simulink model "gm_HDL_pfc_gold_fi_vnl"  (R2024b)
settings: Solver=FixedStepDiscrete  StartTime=0.0  StopTime=.06  RelTol=1e-3
InitFcn:
  | fidelity_pfc_vals;
  | load('C:\Users\angro\Desktop\hil\pfc3ph\matlab\sim\sschdl\pfc_desktop\stateSpaceParameters.mat');
undefined symbols (not defined in the file or in its folder): a, b, c, DiscIntNeverNeededParam, fsw, Gs, s, stateSpaceParameters_1, t_ss, tsw
libraries: simulink x55, hdlmdlgenlib x26, hdlsllib x10, mcbcontrolslib x5, dspsrcs4 x3, slpidlib x2, hdlssclib x2, spsSVPWMGenerator2LevelLib x1, spsPLL3phLib x1
(part 1 of 4)
settings Model: Creator=angro  LastModifiedBy=angro
settings OptimizationCC: BlockReduction=off  ConditionallyExecuteInputs=off  DefaultParameterBehavior=Inlined  InheritOutputTypeSmallerThanSingle=on
settings DebuggingCC: SignalRangeChecking=warning  AlgebraicLoopMsg=error  ArtificialAlgebraicLoopMsg=error  InheritedTsInSrcMsg=none  SingleTaskRateTransMsg=error  UnconnectedInputMsg=warning  UnconnectedOutputMsg=warning  UnconnectedLineMsg=warning
settings HardwareCC: ProdBitPerPointer=32  ProdBitPerSizeT=32  ProdBitPerPtrDiffT=32  ProdLargestAtomicFloat=None  ProdIntDivRoundTo=Undefined  ProdEndianess=Unspecified  ProdWordSize=32  ProdHWDeviceType=ASIC/FPGA->ASIC/FPGA  TargetBitPerPointer=64  TargetBitPerSizeT=64  TargetBitPerPtrDiffT=64  TargetLongLongMode=on  TargetIntDivRoundTo=Zero  TargetEndianess=LittleEndian  TargetWordSize=64  TargetHWDeviceType=Custom Processor->MATLAB Host Computer  ProdEqTarget=off

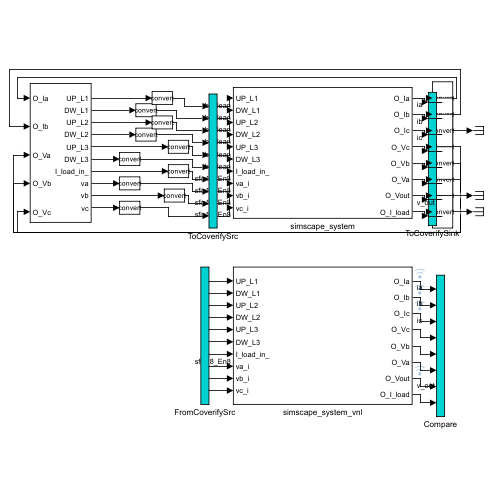
[thumbnail: Simulink's stored preview of the top-level diagram]
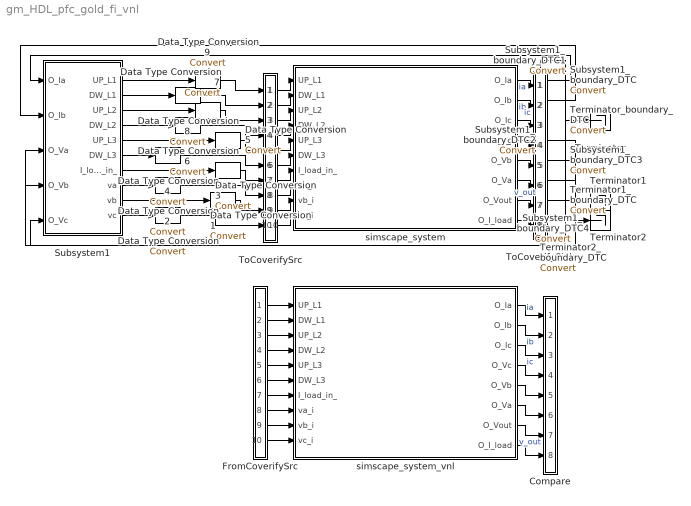
== system gm_HDL_pfc_gold_fi_vnl ==
  Compare : Subsystem
      mask Display: disp('')
  Data Type Conversion{,1..9} (10 alike) : DataTypeConversion  SaturateOnIntegerOverflow=off  RndMeth=Floor
  FromCoverifySrc : Subsystem
      mask Display: disp('')
  Subsystem1 : Subsystem
  Subsystem1_boundary_DTC{,1..4} (5 alike) : DataTypeConversion
  Terminator : Terminator
  Terminator1 : Terminator
  Terminator1_boundary_DTC : DataTypeConversion
  Terminator2 : Terminator
  Terminator2_boundary_DTC : DataTypeConversion
  Terminator_boundary_DTC : DataTypeConversion
  ToCoverifySink : Subsystem
      mask Display: disp('')
  ToCoverifySrc : Subsystem
      mask Display: disp('')
  simscape_system : Subsystem
  simscape_system_vnl : Subsystem
  wires:
  Subsystem1/7(I_load_in_) -> Data Type Conversion3/1
  Subsystem1/1(UP_L1) -> Data Type Conversion9/1
  Subsystem1/2(DW_L1) -> Data Type Conversion8/1
  Subsystem1/3(UP_L2) -> Data Type Conversion7/1
  Subsystem1/4(DW_L2) -> Data Type Conversion6/1
  Subsystem1/5(UP_L3) -> Data Type Conversion5/1
  Subsystem1/6(DW_L3) -> Data Type Conversion4/1
  Subsystem1/8(va) -> Data Type Conversion2/1
  Subsystem1/9(vb) -> Data Type Conversion1/1
  Subsystem1/10(vc) -> Data Type Conversion/1
  Subsystem1_boundary_DTC/1 -> Subsystem1/1(O_Ia)
  Subsystem1_boundary_DTC1/1 -> Subsystem1/2(O_Ib)
  Terminator_boundary_DTC/1 -> Terminator/1
  Subsystem1_boundary_DTC2/1 -> Subsystem1/5(O_Vc)
  Subsystem1_boundary_DTC3/1 -> Subsystem1/4(O_Vb)
  Subsystem1_boundary_DTC4/1 -> Subsystem1/3(O_Va)
  Terminator1_boundary_DTC/1 -> Terminator1/1
  Terminator2_boundary_DTC/1 -> Terminator2/1
  ToCoverifySrc/1(out1) -> simscape_system/1(UP_L1)
  ToCoverifySrc/2(out2) -> simscape_system/2(DW_L1)
  ToCoverifySrc/3(out3) -> simscape_system/3(UP_L2)
  ToCoverifySrc/4(out4) -> simscape_system/4(DW_L2)
  ToCoverifySrc/5(out5) -> simscape_system/5(UP_L3)
  ToCoverifySrc/6(out6) -> simscape_system/6(DW_L3)
  ToCoverifySrc/7(out7) -> simscape_system/7(I_load_in_)
  ToCoverifySrc/8(out8) -> simscape_system/8(va_i)
  ToCoverifySrc/9(out9) -> simscape_system/9(vb_i)
  ToCoverifySrc/10(out10) -> simscape_system/10(vc_i)
  simscape_system/1(O_Ia) -> ToCoverifySink/1(in1)  "ia"
  simscape_system/2(O_Ib) -> ToCoverifySink/2(in2)  "ib"
  simscape_system/3(O_Ic) -> ToCoverifySink/3(in3)  "ic"
  simscape_system/4(O_Vc) -> ToCoverifySink/4(in4)
  simscape_system/5(O_Vb) -> ToCoverifySink/5(in5)
  simscape_system/6(O_Va) -> ToCoverifySink/6(in6)
  simscape_system/7(O_Vout) -> ToCoverifySink/7(in7)  "v_out"
  simscape_system/8(O_I_load) -> ToCoverifySink/8(in8)
  Data Type Conversion9/1 -> ToCoverifySrc/1(in1)
  Data Type Conversion8/1 -> ToCoverifySrc/2(in2)
  Data Type Conversion7/1 -> ToCoverifySrc/3(in3)
  Data Type Conversion6/1 -> ToCoverifySrc/4(in4)
  Data Type Conversion5/1 -> ToCoverifySrc/5(in5)
  Data Type Conversion4/1 -> ToCoverifySrc/6(in6)
  Data Type Conversion3/1 -> ToCoverifySrc/7(in7)
  Data Type Conversion2/1 -> ToCoverifySrc/8(in8)
  Data Type Conversion1/1 -> ToCoverifySrc/9(in9)
  Data Type Conversion/1 -> ToCoverifySrc/10(in10)
  ToCoverifySink/1(out1) -> Subsystem1_boundary_DTC/1
  ToCoverifySink/2(out2) -> Subsystem1_boundary_DTC1/1
  ToCoverifySink/3(out3) -> Terminator_boundary_DTC/1
  ToCoverifySink/4(out4) -> Subsystem1_boundary_DTC2/1
  ToCoverifySink/5(out5) -> Subsystem1_boundary_DTC3/1
  ToCoverifySink/6(out6) -> Subsystem1_boundary_DTC4/1
  ToCoverifySink/7(out7) -> Terminator1_boundary_DTC/1
  ToCoverifySink/8(out8) -> Terminator2_boundary_DTC/1
  FromCoverifySrc/1(out1) -> simscape_system_vnl/1(UP_L1)
  FromCoverifySrc/2(out2) -> simscape_system_vnl/2(DW_L1)
  FromCoverifySrc/3(out3) -> simscape_system_vnl/3(UP_L2)
  FromCoverifySrc/4(out4) -> simscape_system_vnl/4(DW_L2)
  FromCoverifySrc/5(out5) -> simscape_system_vnl/5(UP_L3)
  FromCoverifySrc/6(out6) -> simscape_system_vnl/6(DW_L3)
  FromCoverifySrc/7(out7) -> simscape_system_vnl/7(I_load_in_)
  FromCoverifySrc/8(out8) -> simscape_system_vnl/8(va_i)
  FromCoverifySrc/9(out9) -> simscape_system_vnl/9(vb_i)
  FromCoverifySrc/10(out10) -> simscape_system_vnl/10(vc_i)
  simscape_system_vnl/1(O_Ia) -> Compare/1(in1)  "ia"
  simscape_system_vnl/2(O_Ib) -> Compare/2(in2)  "ib"
  simscape_system_vnl/3(O_Ic) -> Compare/3(in3)  "ic"
  simscape_system_vnl/4(O_Vc) -> Compare/4(in4)
  simscape_system_vnl/5(O_Vb) -> Compare/5(in5)
  simscape_system_vnl/6(O_Va) -> Compare/6(in6)
  simscape_system_vnl/7(O_Vout) -> Compare/7(in7)  "v_out"
  simscape_system_vnl/8(O_I_load) -> Compare/8(in8)

== system gm_HDL_pfc_gold_fi_vnl/Compare ==
  in1 : Inport
  in2 : Inport  Port=2
  in3 : Inport  Port=3
  in4 : Inport  Port=4
  in5 : Inport  Port=5
  in6 : Inport  Port=6
  in7 : Inport  Port=7
  in8 : Inport  Port=8
  Assert_O_I_load : Subsystem
  Assert_O_Ia : Subsystem
  Assert_O_Ib : Subsystem
  Assert_O_Ic : Subsystem
  Assert_O_Va : Subsystem
  Assert_O_Vb : Subsystem
  Assert_O_Vc : Subsystem
  Assert_O_Vout : Subsystem
  CleanupScopes : Subsystem
      settings: OpenFcn=|
      | blkName = gcb; %self block
      | idx = regexp(blkName, '/CleanupScopes$', 'once');
      | blkParent = blkName(1:idx-1);
      | blks=find_system(blkParent, 'LookUnderMasks', 'all','blocktype', 'Scope');
      | for itr = 1:length(blks)
      | 	 hScopeCfg = get_param(blks{itr},'ScopeConfiguration');
      | 	 hScopeCfg.Visible = ~ hScopeCfg.Visible;
      | end
      | drawnow;
      mask Display: fprintf(message('hdlcoder:cosim:vnl_dblclick').getString());
  Enable : Subsystem
      settings: OpenFcn=|
      | blkName = gcb;
      | idx = regexp(blkName, '/Enable$', 'once');
      | blkParent = blkName(1:idx-1);
      | blks=find_system(blkParent, 'LookUnderMasks', 'all','blocktype', 'Assertion');
      | e = get_param(blks{1}, 'Enabled');
      | if strcmp(e, 'on'), f= 'off';, else, f = 'on';, end
      | for ii=1:length(blks), set_param(blks{ii}, 'Enabled', f);, end
      | set_param(gcb, 'MaskDisplay',['fprintf(message(''hdlcoder:cosim:vnl_dblclick_assertions'',','''',upper(e),'''',').getString())']);
      mask Display: fprintf(message('hdlcoder:cosim:vnl_dblclick_assertions','OFF').getString());
  pathdelay{1..8} (8 alike) : Delay  DelayLength=1
  wires:
  in1/1 -> pathdelay1/1
  pathdelay1/1 -> Assert_O_Ia/1(cosim)
  [out1] -> Assert_O_Ia/2(dut)
  in2/1 -> pathdelay2/1
  pathdelay2/1 -> Assert_O_Ib/1(cosim)
  [out2] -> Assert_O_Ib/2(dut)
  in3/1 -> pathdelay3/1
  pathdelay3/1 -> Assert_O_Ic/1(cosim)
  [out3] -> Assert_O_Ic/2(dut)
  in4/1 -> pathdelay4/1
  pathdelay4/1 -> Assert_O_Vc/1(cosim)
  [out4] -> Assert_O_Vc/2(dut)
  in5/1 -> pathdelay5/1
  pathdelay5/1 -> Assert_O_Vb/1(cosim)
  [out5] -> Assert_O_Vb/2(dut)
  in6/1 -> pathdelay6/1
  pathdelay6/1 -> Assert_O_Va/1(cosim)
  [out6] -> Assert_O_Va/2(dut)
  in7/1 -> pathdelay7/1
  pathdelay7/1 -> Assert_O_Vout/1(cosim)
  [out7] -> Assert_O_Vout/2(dut)
  in8/1 -> pathdelay8/1
  pathdelay8/1 -> Assert_O_I_load/1(cosim)
  [out8] -> Assert_O_I_load/2(dut)

== system gm_HDL_pfc_gold_fi_vnl/FromCoverifySrc ==
  out1 : Outport
  out2 : Outport  Port=2
  out3 : Outport  Port=3
  out4 : Outport  Port=4
  out5 : Outport  Port=5
  out6 : Outport  Port=6
  out7 : Outport  Port=7
  out8 : Outport  Port=8
  out9 : Outport  Port=9
  out10 : Outport  Port=10
  wires:
  [in1] -> out1/1
  [in2] -> out2/1
  [in3] -> out3/1
  [in4] -> out4/1
  [in5] -> out5/1
  [in6] -> out6/1
  [in7] -> out7/1
  [in8] -> out8/1
  [in9] -> out9/1
  [in10] -> out10/1

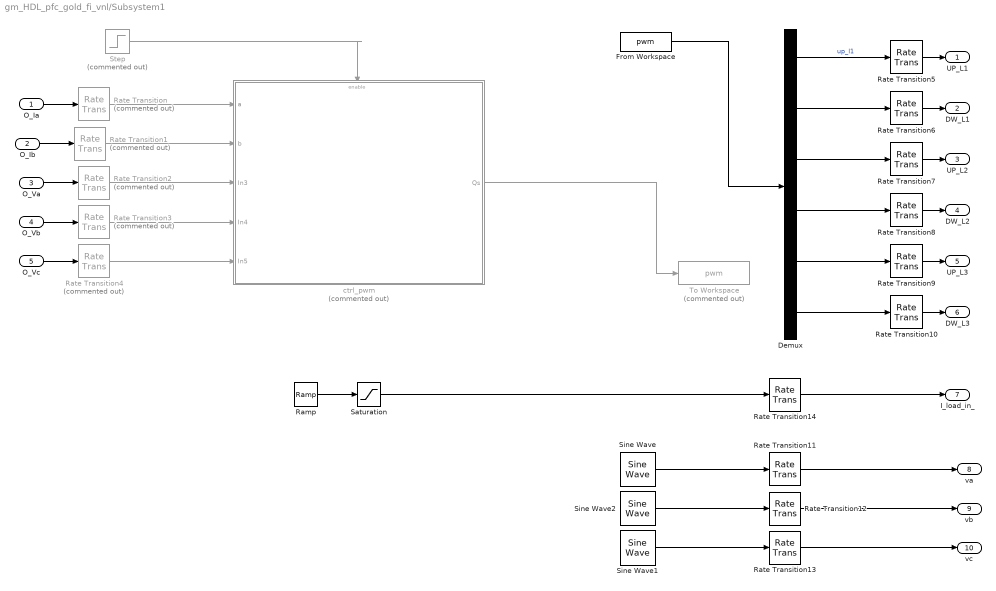
== system gm_HDL_pfc_gold_fi_vnl/Subsystem1 ==
  O_Ia : Inport
  O_Ib : Inport  Port=2
  O_Va : Inport  Port=3
  O_Vb : Inport  Port=4
  O_Vc : Inport  Port=5
  Demux : Demux  Outputs=6
  From Workspace : FromWorkspace  VariableName=pwm  SampleTime=t_ss  Interpolate=off  ZeroCross=off  OutputAfterFinalValue=Holding final value
  Ramp : simulink/Sources/Ramp  slope=1/50  start=2/50  InitialOutput=0
  Rate Transition{,1..4} (5 alike) : RateTransition  Commented=on  OutPortSampleTime=t_ss
  Rate Transition{5..10,14} (7 alike) : RateTransition  OutPortSampleTime=t_ss
  Rate Transition11 : RateTransition
  Rate Transition12 : RateTransition
  Rate Transition13 : RateTransition
  Saturation : Saturate  UpperLimit=2
  Sine Wave : dspsrcs4/Sine Wave  Amplitude=325  Frequency=50  Phase=0  SampleMode=Discrete  OutComplex=Real  CompMethod=Table lookup  TableSize=Speed  SampleTime=tsw  SamplesPerFrame=1  ResetState=Restart at time zero  OutputFrames=off  dataType=double  wordLen=16  udDataType=sfix(16)  fracBitsMode=Best precision  numFracBits=15  OutDataTypeStr=double  LastOutDataTypeStr=double
  Sine Wave1 : dspsrcs4/Sine Wave  Amplitude=325  Frequency=50  Phase=2*pi/3  SampleMode=Discrete  OutComplex=Real  CompMethod=Table lookup  TableSize=Speed  SampleTime=tsw  SamplesPerFrame=1  ResetState=Restart at time zero  OutputFrames=off  dataType=double  wordLen=16  udDataType=sfix(16)  fracBitsMode=Best precision  numFracBits=15  OutDataTypeStr=double  LastOutDataTypeStr=double
  Sine Wave2 : dspsrcs4/Sine Wave  Amplitude=325  Frequency=50  Phase=-2*pi/3  SampleMode=Discrete  OutComplex=Real  CompMethod=Table lookup  TableSize=Speed  SampleTime=tsw  SamplesPerFrame=1  ResetState=Restart at time zero  OutputFrames=off  dataType=double  wordLen=16  udDataType=sfix(16)  fracBitsMode=Best precision  numFracBits=15  OutDataTypeStr=double  LastOutDataTypeStr=double
  Step : Step  Commented=on  Time=2/50  SampleTime=0
  To Workspace : ToWorkspace  Commented=on  VariableName=pwm  SaveFormat=Timeseries  SampleTime=-1
  ctrl_pwm : Subsystem  Commented=on
  UP_L1 : Outport
  DW_L1 : Outport  Port=2
  UP_L2 : Outport  Port=3
  DW_L2 : Outport  Port=4
  UP_L3 : Outport  Port=5
  DW_L3 : Outport  Port=6
  I_load_in_ : Outport  Port=7
  va : Outport  Port=8
  vb : Outport  Port=9
  vc : Outport  Port=10
  wires:
  Demux/5 -> Rate Transition9/1
  Demux/1 -> Rate Transition5/1  "up_l1"
  Demux/6 -> Rate Transition10/1
  Demux/4 -> Rate Transition8/1
  Demux/3 -> Rate Transition7/1
  Demux/2 -> Rate Transition6/1
  O_Ia/1 -> Rate Transition/1
  O_Ib/1 -> Rate Transition1/1
  O_Va/1 -> Rate Transition2/1
  O_Vb/1 -> Rate Transition3/1
  O_Vc/1 -> Rate Transition4/1
  Rate Transition5/1 -> UP_L1/1
  Rate Transition6/1 -> DW_L1/1
  Rate Transition7/1 -> UP_L2/1
  Rate Transition8/1 -> DW_L2/1
  Rate Transition9/1 -> UP_L3/1
  Rate Transition10/1 -> DW_L3/1
  Saturation/1 -> Rate Transition14/1
  Sine Wave/1 -> Rate Transition11/1
  Sine Wave2/1 -> Rate Transition12/1
  Sine Wave1/1 -> Rate Transition13/1
  Rate Transition11/1 -> va/1
  Rate Transition12/1 -> vb/1
  Rate Transition13/1 -> vc/1
  ctrl_pwm/1(Qs) -> To Workspace/1
  Rate Transition/1 -> ctrl_pwm/1(a)
  Rate Transition1/1 -> ctrl_pwm/2(b)
  Rate Transition2/1 -> ctrl_pwm/3(In3)
  Rate Transition3/1 -> ctrl_pwm/4(In4)
  Rate Transition4/1 -> ctrl_pwm/5(In5)
  Step/1 -> ctrl_pwm/Enable
  Rate Transition14/1 -> I_load_in_/1
  Ramp/1 -> Saturation/1
  From Workspace/1 -> Demux/1

== system gm_HDL_pfc_gold_fi_vnl/ToCoverifySink ==
  in1 : Inport
  in2 : Inport  Port=2
  in3 : Inport  Port=3
  in4 : Inport  Port=4
  in5 : Inport  Port=5
  in6 : Inport  Port=6
  in7 : Inport  Port=7
  in8 : Inport  Port=8
  out1 : Outport
  out2 : Outport  Port=2
  out3 : Outport  Port=3
  out4 : Outport  Port=4
  out5 : Outport  Port=5
  out6 : Outport  Port=6
  out7 : Outport  Port=7
  out8 : Outport  Port=8
  tag scope: out1=global, out2=global, out3=global, out4=global, out5=global, out6=global, out7=global, out8=global
  wires:
  in1/1 -> out1/1, [out1]
  in2/1 -> out2/1, [out2]
  in3/1 -> out3/1, [out3]
  in4/1 -> out4/1, [out4]
  in5/1 -> out5/1, [out5]
  in6/1 -> out6/1, [out6]
  in7/1 -> out7/1, [out7]
  in8/1 -> out8/1, [out8]

== system gm_HDL_pfc_gold_fi_vnl/ToCoverifySrc ==
  in1 : Inport
  in2 : Inport  Port=2
  in3 : Inport  Port=3
  in4 : Inport  Port=4
  in5 : Inport  Port=5
  in6 : Inport  Port=6
  in7 : Inport  Port=7
  in8 : Inport  Port=8
  in9 : Inport  Port=9
  in10 : Inport  Port=10
  out1 : Outport
  out2 : Outport  Port=2
  out3 : Outport  Port=3
  out4 : Outport  Port=4
  out5 : Outport  Port=5
  out6 : Outport  Port=6
  out7 : Outport  Port=7
  out8 : Outport  Port=8
  out9 : Outport  Port=9
  out10 : Outport  Port=10
  tag scope: in10=global, in1=global, in2=global, in3=global, in4=global, in5=global, in6=global, in7=global, in8=global, in9=global
  wires:
  in1/1 -> out1/1, [in1]
  in2/1 -> out2/1, [in2]
  in3/1 -> out3/1, [in3]
  in4/1 -> out4/1, [in4]
  in5/1 -> out5/1, [in5]
  in6/1 -> out6/1, [in6]
  in7/1 -> out7/1, [in7]
  in8/1 -> out8/1, [in8]
  in9/1 -> out9/1, [in9]
  in10/1 -> out10/1, [in10]

== system gm_HDL_pfc_gold_fi_vnl/simscape_system ==
  UP_L1 : Inport  OutDataTypeStr=boolean  PortDimensions=1  SampleTime=5.12820512820513e-07
  DW_L1 : Inport  Port=2  OutDataTypeStr=boolean  PortDimensions=1  SampleTime=5.12820512820513e-07
  UP_L2 : Inport  Port=3  OutDataTypeStr=boolean  PortDimensions=1  SampleTime=5.12820512820513e-07
  DW_L2 : Inport  Port=4  OutDataTypeStr=boolean  PortDimensions=1  SampleTime=5.12820512820513e-07
  UP_L3 : Inport  Port=5  OutDataTypeStr=boolean  PortDimensions=1  SampleTime=5.12820512820513e-07
  DW_L3 : Inport  Port=6  OutDataTypeStr=boolean  PortDimensions=1  SampleTime=5.12820512820513e-07
  I_load_in_ : Inport  Port=7  OutDataTypeStr=fixdt(1, 18, 8)  PortDimensions=1  SampleTime=5.12820512820513e-07
  va_i : Inport  Port=8  OutDataTypeStr=fixdt(1, 18, 8)  PortDimensions=1  SampleTime=5.12820512820513e-07  LockScale=on
  vb_i : Inport  Port=9  OutDataTypeStr=fixdt(1, 18, 8)  PortDimensions=1  SampleTime=5.12820512820513e-07  LockScale=on
  vc_i : Inport  Port=10  OutDataTypeStr=fixdt(1, 18, 8)  PortDimensions=1  SampleTime=5.12820512820513e-07  LockScale=on
  FET_CTRL : Subsystem
  HDL Subsystem : Subsystem
  Rate Transition{1..10} (10 alike) : hdlmdlgenlib/Buffer
  concatenate : Concatenate  NumInputs=6
  concatenate1 : Concatenate  NumInputs=6
  concatenate2 : Concatenate  NumInputs=6
  ctr_0_36 : hdlsllib/Sources/HDL Counter  CountType=Count limited  CountInit=double(0)  CountStep=double(1)  CountMax=double(36)  CountFromType=Initial value  CountFrom=double(0)  CountResetPort=off  CountLoadPort=off  CountEnbPort=off  CountDirPort=off  CountHitOutputPort=off  CountDataType=Unsigned  CountWordLen=6  CountFracLen=0  CountSampTime=1.38600138600139e-08
  t : Demux  Outputs=6
  O_Ia : Outport  SampleTime=5.12820512820513e-07
  O_Ib : Outport  Port=2  SampleTime=5.12820512820513e-07
  O_Ic : Outport  Port=3  SampleTime=5.12820512820513e-07
  O_Vc : Outport  Port=4  SampleTime=5.12820512820513e-07
  O_Vb : Outport  Port=5  SampleTime=5.12820512820513e-07
  O_Va : Outport  Port=6  SampleTime=5.12820512820513e-07
  O_Vout : Outport  Port=7  SampleTime=5.12820512820513e-07
  O_I_load : Outport  Port=8  SampleTime=5.12820512820513e-07
  wires:
  FET_CTRL/1(ic) -> t/1
  DW_L2/1 -> concatenate/3
  HDL Subsystem/20(Va) -> O_Va/1
  HDL Subsystem/19(Vc) -> O_Vc/1
  DW_L3/1 -> concatenate/4
  HDL Subsystem/18(Vb) -> O_Vb/1
  HDL Subsystem/16(Ic) -> O_Ic/1
  HDL Subsystem/15(Ib) -> O_Ib/1
  HDL Subsystem/14(Vout) -> O_Vout/1
  HDL Subsystem/11(vs_out_MOSFET4) -> concatenate2/6
  UP_L2/1 -> concatenate/6
  HDL Subsystem/9(vs_out_MOSFET3) -> concatenate2/4
  concatenate1/1 -> FET_CTRL/2(is)
  HDL Subsystem/8(is_out_MOSFET3) -> concatenate1/4
  HDL Subsystem/7(vs_out_MOSFET2) -> concatenate2/3
  HDL Subsystem/6(is_out_MOSFET2) -> concatenate1/3
  UP_L3/1 -> concatenate/5
  HDL Subsystem/5(vs_out_MOSFET1) -> concatenate2/2
  HDL Subsystem/4(is_out_MOSFET1) -> concatenate1/2
  HDL Subsystem/3(vs_out_MOSFET) -> concatenate2/1
  HDL Subsystem/2(is_out_MOSFET) -> concatenate1/1
  HDL Subsystem/1(I_load) -> O_I_load/1
  ctr_0_36/1 -> FET_CTRL/4(sch_ctr_36), HDL Subsystem/11(sch_ctr_36)
  HDL Subsystem/17(Ia) -> O_Ia/1
  concatenate2/1 -> FET_CTRL/1(vs)
  Rate Transition6/1 -> HDL Subsystem/10(vc)
  HDL Subsystem/13(vs_out_MOSFET5) -> concatenate2/5
  Rate Transition1/1 -> HDL Subsystem/1(I_load_in)
  Rate Transition3/1 -> HDL Subsystem/9(vb)
  Rate Transition8/1 -> HDL Subsystem/6(ic_in_MOSFET4)
  Rate Transition9/1 -> HDL Subsystem/7(ic_in_MOSFET5)
  Rate Transition5/1 -> HDL Subsystem/5(ic_in_MOSFET3)
  Rate Transition4/1 -> HDL Subsystem/4(ic_in_MOSFET2)
  HDL Subsystem/10(is_out_MOSFET4) -> concatenate1/6
  Rate Transition7/1 -> HDL Subsystem/2(ic_in_MOSFET)
  Rate Transition10/1 -> HDL Subsystem/3(ic_in_MOSFET1)
  vc_i/1 -> Rate Transition6/1
  Rate Transition2/1 -> HDL Subsystem/8(va)
  DW_L1/1 -> concatenate/2
  vb_i/1 -> Rate Transition3/1
  UP_L1/1 -> concatenate/1
  I_load_in_/1 -> Rate Transition1/1
  t/6 -> Rate Transition8/1
  t/5 -> Rate Transition9/1
  t/4 -> Rate Transition5/1
  t/3 -> Rate Transition4/1
  HDL Subsystem/12(is_out_MOSFET5) -> concatenate1/5
  concatenate/1 -> FET_CTRL/3(G)
  va_i/1 -> Rate Transition2/1
  t/2 -> Rate Transition10/1
  t/1 -> Rate Transition7/1

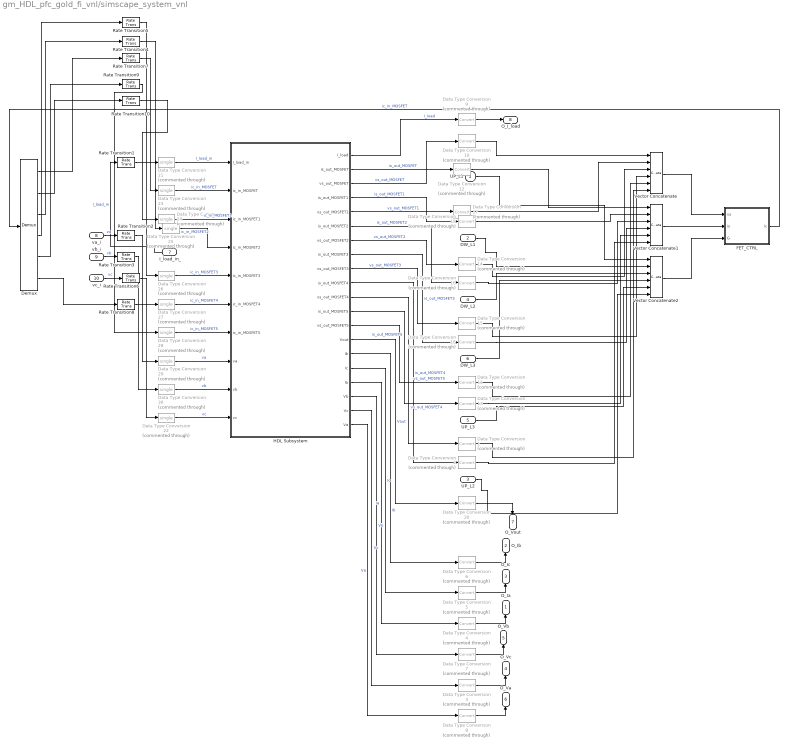
== system gm_HDL_pfc_gold_fi_vnl/simscape_system_vnl ==
  UP_L1 : Inport
  DW_L1 : Inport  Port=2
  UP_L2 : Inport  Port=3
  DW_L2 : Inport  Port=4
  UP_L3 : Inport  Port=5
  DW_L3 : Inport  Port=6
  I_load_in_ : Inport  Port=7  OutDataTypeStr=fixdt(1,18,8)
  va_i : Inport  Port=8  LockScale=on
  vb_i : Inport  Port=9  LockScale=on
  vc_i : Inport  Port=10  LockScale=on
  Data Type Conversion{1..20} (20 alike) : DataTypeConversion  Commented=through  RndMeth=Nearest  SaturateOnIntegerOverflow=off  LockScale=on
  Data Type Conversion{21..30} (10 alike) : DataTypeConversion  Commented=through  OutDataTypeStr=single  RndMeth=Nearest  SaturateOnIntegerOverflow=off
  Demux : Demux  Outputs=6
  FET_CTRL : Subsystem
  HDL Subsystem : Subsystem
  Rate Transition{1..10} (10 alike) : RateTransition  OutPortSampleTime=t_ss
  Vector Concatenate : Concatenate  NumInputs=6
  Vector Concatenate1 : Concatenate  NumInputs=6
  Vector Concatenate2 : Concatenate  NumInputs=6
  O_Ia : Outport
  O_Ib : Outport  Port=2
  O_Ic : Outport  Port=3
  O_Vc : Outport  Port=4
  O_Vb : Outport  Port=5
  O_Va : Outport  Port=6
  O_Vout : Outport  Port=7
  O_I_load : Outport  Port=8
  wires:
  FET_CTRL/1(ic) -> Demux/1  "ic_in_MOSFET"
  Demux/6 -> Rate Transition8/1
  Demux/5 -> Rate Transition9/1
  Demux/4 -> Rate Transition5/1
  Demux/3 -> Rate Transition4/1
  Demux/2 -> Rate Transition10/1
  Demux/1 -> Rate Transition7/1
  Vector Concatenate2/1 -> FET_CTRL/3(G)
  Vector Concatenate1/1 -> FET_CTRL/2(is)
  Vector Concatenate/1 -> FET_CTRL/1(vs)
  Data Type Conversion3/1 -> O_Vc/1
  Data Type Conversion7/1 -> O_Vb/1
  Data Type Conversion4/1 -> O_Ia/1
  Data Type Conversion5/1 -> O_Ic/1
  Data Type Conversion6/1 -> O_Ib/1
  Data Type Conversion1/1 -> Vector Concatenate/6
  Data Type Conversion11/1 -> Vector Concatenate/5
  Data Type Conversion19/1 -> Vector Concatenate1/2
  Data Type Conversion17/1 -> Vector Concatenate/2
  UP_L1/1 -> Vector Concatenate2/1
  DW_L1/1 -> Vector Concatenate2/2
  Data Type Conversion10/1 -> Vector Concatenate/1
  Data Type Conversion13/1 -> Vector Concatenate1/5
  Data Type Conversion9/1 -> O_I_load/1
  HDL Subsystem/20(Va) -> Data Type Conversion8/1  "Va"
  HDL Subsystem/19(Vc) -> Data Type Conversion3/1  "Vc"
  HDL Subsystem/18(Vb) -> Data Type Conversion7/1  "Vb"
  HDL Subsystem/17(Ia) -> Data Type Conversion4/1  "Ia"
  HDL Subsystem/16(Ic) -> Data Type Conversion5/1  "Ic"
  HDL Subsystem/15(Ib) -> Data Type Conversion6/1  "Ib"
  Data Type Conversion15/1 -> Vector Concatenate/4
  HDL Subsystem/14(Vout) -> Data Type Conversion20/1  "Vout"
  HDL Subsystem/13(vs_out_MOSFET5) -> Data Type Conversion11/1  "vs_out_MOSFET5"
  HDL Subsystem/12(is_out_MOSFET5) -> Data Type Conversion13/1  "is_out_MOSFET5"
  HDL Subsystem/9(vs_out_MOSFET3) -> Data Type Conversion15/1  "vs_out_MOSFET3"
  HDL Subsystem/7(vs_out_MOSFET2) -> Data Type Conversion14/1  "vs_out_MOSFET2"
  HDL Subsystem/6(is_out_MOSFET2) -> Data Type Conversion16/1  "is_out_MOSFET2"
  HDL Subsystem/5(vs_out_MOSFET1) -> Data Type Conversion17/1  "vs_out_MOSFET1"
  HDL Subsystem/4(is_out_MOSFET1) -> Data Type Conversion19/1  "is_out_MOSFET1"
  HDL Subsystem/3(vs_out_MOSFET) -> Data Type Conversion10/1  "vs_out_MOSFET"
  HDL Subsystem/1(I_load) -> Data Type Conversion9/1  "I_load"
  Data Type Conversion30/1 -> HDL Subsystem/9(vb)  "vb"
  HDL Subsystem/8(is_out_MOSFET3) -> Data Type Conversion18/1  "is_out_MOSFET3"
  Data Type Conversion29/1 -> HDL Subsystem/8(va)  "va"
  Data Type Conversion28/1 -> HDL Subsystem/7(ic_in_MOSFET5)  "ic_in_MOSFET5"
  Data Type Conversion27/1 -> HDL Subsystem/6(ic_in_MOSFET4)  "ic_in_MOSFET4"
  Data Type Conversion14/1 -> Vector Concatenate/3
  Data Type Conversion24/1 -> HDL Subsystem/3(ic_in_MOSFET1)  "ic_in_MOSFET1"
  HDL Subsystem/10(is_out_MOSFET4) -> Data Type Conversion2/1  "is_out_MOSFET4"
  Data Type Conversion23/1 -> HDL Subsystem/2(ic_in_MOSFET)  "ic_in_MOSFET"
  Data Type Conversion20/1 -> O_Vout/1
  Data Type Conversion21/1 -> HDL Subsystem/1(I_load_in)  "I_load_in"
  Rate Transition8/1 -> Data Type Conversion27/1
  Data Type Conversion8/1 -> O_Va/1
  Rate Transition6/1 -> Data Type Conversion22/1
  Rate Transition3/1 -> Data Type Conversion30/1
  Rate Transition2/1 -> Data Type Conversion29/1
  Rate Transition1/1 -> Data Type Conversion21/1
  HDL Subsystem/11(vs_out_MOSFET4) -> Data Type Conversion1/1  "vs_out_MOSFET4"
  Data Type Conversion16/1 -> Vector Concatenate1/3
  Rate Transition9/1 -> Data Type Conversion28/1
  Rate Transition7/1 -> Data Type Conversion23/1
  Data Type Conversion18/1 -> Vector Concatenate1/4
  Data Type Conversion26/1 -> HDL Subsystem/5(ic_in_MOSFET3)  "ic_in_MOSFET3"
  Data Type Conversion2/1 -> Vector Concatenate1/6
  Data Type Conversion22/1 -> HDL Subsystem/10(vc)  "vc"
  Rate Transition4/1 -> Data Type Conversion25/1
  Rate Transition5/1 -> Data Type Conversion26/1
  vb_i/1 -> Rate Transition3/1  "vb"
  UP_L3/1 -> Vector Concatenate2/5
  UP_L2/1 -> Vector Concatenate2/6
  I_load_in_/1 -> Rate Transition1/1  "I_load_in"
  vc_i/1 -> Rate Transition6/1  "vc"
  HDL Subsystem/2(is_out_MOSFET) -> Data Type Conversion12/1  "is_out_MOSFET"
  Data Type Conversion12/1 -> Vector Concatenate1/1
  DW_L2/1 -> Vector Concatenate2/3
  va_i/1 -> Rate Transition2/1  "va"
  DW_L3/1 -> Vector Concatenate2/4
  Rate Transition10/1 -> Data Type Conversion24/1
  Data Type Conversion25/1 -> HDL Subsystem/4(ic_in_MOSFET2)  "ic_in_MOSFET2"

== system gm_HDL_pfc_gold_fi_vnl/Compare/Assert_O_I_load ==
  cosim : Inport
  dut : Inport  Port=2
  AssertEq : Assertion  StopWhenAssertionFail=off
  Compare To Zero : simulink/Logic and Bit Operations/Compare To Zero  relop===  OutDataTypeStr=boolean
  Constant1 : Constant  Value=0  OutDataTypeStr=Inherit: Inherit via back propagation  SampleTime=-1
  Counter : simulink/Sources/Counter Free-Running  NumBits=32  tsamp=-1
  IgnoreCycles : Constant  Value=2  OutDataTypeStr=Inherit: Inherit via back propagation  SampleTime=-1
  Relational Operator : RelationalOperator  Operator=<  OutDataTypeStr=boolean  InputSameDT=off
  Relational Operator1 : RelationalOperator  Operator===  OutDataTypeStr=boolean  InputSameDT=off
  Switch : Switch  Criteria=u2 ~= 0  SaturateOnIntegerOverflow=off  InputSameDT=off
  Switch1 : Switch  Criteria=u2 ~= 0  SaturateOnIntegerOverflow=off  InputSameDT=off
  compare: O_I_load : Scope  NumInputPorts=3
  wires:
  Compare To Zero/1 -> compare: O_I_load/3  "err"
  Relational Operator1/1 -> Compare To Zero/1, AssertEq/1
  Switch1/1 -> compare: O_I_load/1, Relational Operator1/1
  Switch/1 -> compare: O_I_load/2, Relational Operator1/2
  Constant1/1 -> Switch/1, Switch1/1
  Relational Operator/1 -> Switch/2, Switch1/2
  cosim/1 -> Switch1/3  "cosim"
  dut/1 -> Switch/3  "dut ref"
  Counter/1 -> Relational Operator/1
  IgnoreCycles/1 -> Relational Operator/2

== system gm_HDL_pfc_gold_fi_vnl/Compare/Assert_O_Ia ==
  cosim : Inport
  dut : Inport  Port=2
  AssertEq : Assertion  StopWhenAssertionFail=off
  Compare To Zero : simulink/Logic and Bit Operations/Compare To Zero  relop===  OutDataTypeStr=boolean
  Constant1 : Constant  Value=0  OutDataTypeStr=Inherit: Inherit via back propagation  SampleTime=-1
  Counter : simulink/Sources/Counter Free-Running  NumBits=32  tsamp=-1
  IgnoreCycles : Constant  Value=2  OutDataTypeStr=Inherit: Inherit via back propagation  SampleTime=-1
  Relational Operator : RelationalOperator  Operator=<  OutDataTypeStr=boolean  InputSameDT=off
  Relational Operator1 : RelationalOperator  Operator===  OutDataTypeStr=boolean  InputSameDT=off
  Switch : Switch  Criteria=u2 ~= 0  SaturateOnIntegerOverflow=off  InputSameDT=off
  Switch1 : Switch  Criteria=u2 ~= 0  SaturateOnIntegerOverflow=off  InputSameDT=off
  compare: O_Ia : Scope  NumInputPorts=3
  wires:
  Compare To Zero/1 -> compare: O_Ia/3  "err"
  Relational Operator1/1 -> Compare To Zero/1, AssertEq/1
  Switch1/1 -> compare: O_Ia/1, Relational Operator1/1
  Switch/1 -> compare: O_Ia/2, Relational Operator1/2
  Constant1/1 -> Switch/1, Switch1/1
  Relational Operator/1 -> Switch/2, Switch1/2
  cosim/1 -> Switch1/3  "cosim"
  dut/1 -> Switch/3  "dut ref"
  Counter/1 -> Relational Operator/1
  IgnoreCycles/1 -> Relational Operator/2

== system gm_HDL_pfc_gold_fi_vnl/Compare/Assert_O_Ib ==
  cosim : Inport
  dut : Inport  Port=2
  AssertEq : Assertion  StopWhenAssertionFail=off
  Compare To Zero : simulink/Logic and Bit Operations/Compare To Zero  relop===  OutDataTypeStr=boolean
  Constant1 : Constant  Value=0  OutDataTypeStr=Inherit: Inherit via back propagation  SampleTime=-1
  Counter : simulink/Sources/Counter Free-Running  NumBits=32  tsamp=-1
  IgnoreCycles : Constant  Value=2  OutDataTypeStr=Inherit: Inherit via back propagation  SampleTime=-1
  Relational Operator : RelationalOperator  Operator=<  OutDataTypeStr=boolean  InputSameDT=off
  Relational Operator1 : RelationalOperator  Operator===  OutDataTypeStr=boolean  InputSameDT=off
  Switch : Switch  Criteria=u2 ~= 0  SaturateOnIntegerOverflow=off  InputSameDT=off
  Switch1 : Switch  Criteria=u2 ~= 0  SaturateOnIntegerOverflow=off  InputSameDT=off
  compare: O_Ib : Scope  NumInputPorts=3
  wires:
  Compare To Zero/1 -> compare: O_Ib/3  "err"
  Relational Operator1/1 -> Compare To Zero/1, AssertEq/1
  Switch1/1 -> compare: O_Ib/1, Relational Operator1/1
  Switch/1 -> compare: O_Ib/2, Relational Operator1/2
  Constant1/1 -> Switch/1, Switch1/1
  Relational Operator/1 -> Switch/2, Switch1/2
  cosim/1 -> Switch1/3  "cosim"
  dut/1 -> Switch/3  "dut ref"
  Counter/1 -> Relational Operator/1
  IgnoreCycles/1 -> Relational Operator/2

== system gm_HDL_pfc_gold_fi_vnl/Compare/Assert_O_Ic ==
  cosim : Inport
  dut : Inport  Port=2
  AssertEq : Assertion  StopWhenAssertionFail=off
  Compare To Zero : simulink/Logic and Bit Operations/Compare To Zero  relop===  OutDataTypeStr=boolean
  Constant1 : Constant  Value=0  OutDataTypeStr=Inherit: Inherit via back propagation  SampleTime=-1
  Counter : simulink/Sources/Counter Free-Running  NumBits=32  tsamp=-1
  IgnoreCycles : Constant  Value=2  OutDataTypeStr=Inherit: Inherit via back propagation  SampleTime=-1
  Relational Operator : RelationalOperator  Operator=<  OutDataTypeStr=boolean  InputSameDT=off
  Relational Operator1 : RelationalOperator  Operator===  OutDataTypeStr=boolean  InputSameDT=off
  Switch : Switch  Criteria=u2 ~= 0  SaturateOnIntegerOverflow=off  InputSameDT=off
  Switch1 : Switch  Criteria=u2 ~= 0  SaturateOnIntegerOverflow=off  InputSameDT=off
  compare: O_Ic : Scope  NumInputPorts=3
  wires:
  Compare To Zero/1 -> compare: O_Ic/3  "err"
  Relational Operator1/1 -> Compare To Zero/1, AssertEq/1
  Switch1/1 -> compare: O_Ic/1, Relational Operator1/1
  Switch/1 -> compare: O_Ic/2, Relational Operator1/2
  Constant1/1 -> Switch/1, Switch1/1
  Relational Operator/1 -> Switch/2, Switch1/2
  cosim/1 -> Switch1/3  "cosim"
  dut/1 -> Switch/3  "dut ref"
  Counter/1 -> Relational Operator/1
  IgnoreCycles/1 -> Relational Operator/2

== system gm_HDL_pfc_gold_fi_vnl/Compare/Assert_O_Va ==
  cosim : Inport
  dut : Inport  Port=2
  AssertEq : Assertion  StopWhenAssertionFail=off
  Compare To Zero : simulink/Logic and Bit Operations/Compare To Zero  relop===  OutDataTypeStr=boolean
  Constant1 : Constant  Value=0  OutDataTypeStr=Inherit: Inherit via back propagation  SampleTime=-1
  Counter : simulink/Sources/Counter Free-Running  NumBits=32  tsamp=-1
  IgnoreCycles : Constant  Value=2  OutDataTypeStr=Inherit: Inherit via back propagation  SampleTime=-1
  Relational Operator : RelationalOperator  Operator=<  OutDataTypeStr=boolean  InputSameDT=off
  Relational Operator1 : RelationalOperator  Operator===  OutDataTypeStr=boolean  InputSameDT=off
  Switch : Switch  Criteria=u2 ~= 0  SaturateOnIntegerOverflow=off  InputSameDT=off
  Switch1 : Switch  Criteria=u2 ~= 0  SaturateOnIntegerOverflow=off  InputSameDT=off
  compare: O_Va : Scope  NumInputPorts=3
  wires:
  Compare To Zero/1 -> compare: O_Va/3  "err"
  Relational Operator1/1 -> Compare To Zero/1, AssertEq/1
  Switch1/1 -> compare: O_Va/1, Relational Operator1/1
  Switch/1 -> compare: O_Va/2, Relational Operator1/2
  Constant1/1 -> Switch/1, Switch1/1
  Relational Operator/1 -> Switch/2, Switch1/2
  cosim/1 -> Switch1/3  "cosim"
  dut/1 -> Switch/3  "dut ref"
  Counter/1 -> Relational Operator/1
  IgnoreCycles/1 -> Relational Operator/2

== system gm_HDL_pfc_gold_fi_vnl/Compare/Assert_O_Vb ==
  cosim : Inport
  dut : Inport  Port=2
  AssertEq : Assertion  StopWhenAssertionFail=off
  Compare To Zero : simulink/Logic and Bit Operations/Compare To Zero  relop===  OutDataTypeStr=boolean
  Constant1 : Constant  Value=0  OutDataTypeStr=Inherit: Inherit via back propagation  SampleTime=-1
  Counter : simulink/Sources/Counter Free-Running  NumBits=32  tsamp=-1
  IgnoreCycles : Constant  Value=2  OutDataTypeStr=Inherit: Inherit via back propagation  SampleTime=-1
  Relational Operator : RelationalOperator  Operator=<  OutDataTypeStr=boolean  InputSameDT=off
  Relational Operator1 : RelationalOperator  Operator===  OutDataTypeStr=boolean  InputSameDT=off
  Switch : Switch  Criteria=u2 ~= 0  SaturateOnIntegerOverflow=off  InputSameDT=off
  Switch1 : Switch  Criteria=u2 ~= 0  SaturateOnIntegerOverflow=off  InputSameDT=off
  compare: O_Vb : Scope  NumInputPorts=3
  wires:
  Compare To Zero/1 -> compare: O_Vb/3  "err"
  Relational Operator1/1 -> Compare To Zero/1, AssertEq/1
  Switch1/1 -> compare: O_Vb/1, Relational Operator1/1
  Switch/1 -> compare: O_Vb/2, Relational Operator1/2
  Constant1/1 -> Switch/1, Switch1/1
  Relational Operator/1 -> Switch/2, Switch1/2
  cosim/1 -> Switch1/3  "cosim"
  dut/1 -> Switch/3  "dut ref"
  Counter/1 -> Relational Operator/1
  IgnoreCycles/1 -> Relational Operator/2

== system gm_HDL_pfc_gold_fi_vnl/Compare/Assert_O_Vc ==
  cosim : Inport
  dut : Inport  Port=2
  AssertEq : Assertion  StopWhenAssertionFail=off
  Compare To Zero : simulink/Logic and Bit Operations/Compare To Zero  relop===  OutDataTypeStr=boolean
  Constant1 : Constant  Value=0  OutDataTypeStr=Inherit: Inherit via back propagation  SampleTime=-1
  Counter : simulink/Sources/Counter Free-Running  NumBits=32  tsamp=-1
  IgnoreCycles : Constant  Value=2  OutDataTypeStr=Inherit: Inherit via back propagation  SampleTime=-1
  Relational Operator : RelationalOperator  Operator=<  OutDataTypeStr=boolean  InputSameDT=off
  Relational Operator1 : RelationalOperator  Operator===  OutDataTypeStr=boolean  InputSameDT=off
  Switch : Switch  Criteria=u2 ~= 0  SaturateOnIntegerOverflow=off  InputSameDT=off
  Switch1 : Switch  Criteria=u2 ~= 0  SaturateOnIntegerOverflow=off  InputSameDT=off
  compare: O_Vc : Scope  NumInputPorts=3
  wires:
  Compare To Zero/1 -> compare: O_Vc/3  "err"
  Relational Operator1/1 -> Compare To Zero/1, AssertEq/1
  Switch1/1 -> compare: O_Vc/1, Relational Operator1/1
  Switch/1 -> compare: O_Vc/2, Relational Operator1/2
  Constant1/1 -> Switch/1, Switch1/1
  Relational Operator/1 -> Switch/2, Switch1/2
  cosim/1 -> Switch1/3  "cosim"
  dut/1 -> Switch/3  "dut ref"
  Counter/1 -> Relational Operator/1
  IgnoreCycles/1 -> Relational Operator/2

== system gm_HDL_pfc_gold_fi_vnl/Compare/Assert_O_Vout ==
  cosim : Inport
  dut : Inport  Port=2
  AssertEq : Assertion  StopWhenAssertionFail=off
  Compare To Zero : simulink/Logic and Bit Operations/Compare To Zero  relop===  OutDataTypeStr=boolean
  Constant1 : Constant  Value=0  OutDataTypeStr=Inherit: Inherit via back propagation  SampleTime=-1
  Counter : simulink/Sources/Counter Free-Running  NumBits=32  tsamp=-1
  IgnoreCycles : Constant  Value=2  OutDataTypeStr=Inherit: Inherit via back propagation  SampleTime=-1
  Relational Operator : RelationalOperator  Operator=<  OutDataTypeStr=boolean  InputSameDT=off
  Relational Operator1 : RelationalOperator  Operator===  OutDataTypeStr=boolean  InputSameDT=off
  Switch : Switch  Criteria=u2 ~= 0  SaturateOnIntegerOverflow=off  InputSameDT=off
  Switch1 : Switch  Criteria=u2 ~= 0  SaturateOnIntegerOverflow=off  InputSameDT=off
  compare: O_Vout : Scope  NumInputPorts=3
  wires:
  Compare To Zero/1 -> compare: O_Vout/3  "err"
  Relational Operator1/1 -> Compare To Zero/1, AssertEq/1
  Switch1/1 -> compare: O_Vout/1, Relational Operator1/1
  Switch/1 -> compare: O_Vout/2, Relational Operator1/2
  Constant1/1 -> Switch/1, Switch1/1
  Relational Operator/1 -> Switch/2, Switch1/2
  cosim/1 -> Switch1/3  "cosim"
  dut/1 -> Switch/3  "dut ref"
  Counter/1 -> Relational Operator/1
  IgnoreCycles/1 -> Relational Operator/2

== system gm_HDL_pfc_gold_fi_vnl/Compare/CleanupScopes ==

== system gm_HDL_pfc_gold_fi_vnl/Compare/Enable ==

== system gm_HDL_pfc_gold_fi_vnl/Subsystem1/ctrl_pwm ==
  a : Inport
  b : Inport  Port=2
  In3 : Inport  Port=3
  In4 : Inport  Port=4
  In5 : Inport  Port=5
  Enable : EnablePort
  PI_CTRL : Subsystem
  SVPWM : Subsystem
  transforms : Subsystem
  Qs : Outport
  wires:
  transforms/1(id) -> PI_CTRL/1(id)
  transforms/3(angle) -> SVPWM/2(angle)
  PI_CTRL/1(Vd_inductor) -> SVPWM/1(Vd_inductor)
  a/1 -> transforms/1(a)
  In5/1 -> transforms/5(In5)
  transforms/2(iq) -> PI_CTRL/2(iq)
  SVPWM/1(P) -> Qs/1  "Qs"
  PI_CTRL/2(Vq_inductor) -> SVPWM/3(Vq_inductor)
  b/1 -> transforms/2(b)
  In3/1 -> transforms/3(In3)
  In4/1 -> transforms/4(In4)

== system gm_HDL_pfc_gold_fi_vnl/simscape_system/FET_CTRL ==
  vs : Inport  OutDataTypeStr=fixdt(1, 18, 6)  PortDimensions=[6]  SampleTime=1.38600138600139e-08
  is : Inport  Port=2  OutDataTypeStr=fixdt(1, 18, 6)  PortDimensions=[6]  SampleTime=1.38600138600139e-08
  G : Inport  Port=3  OutDataTypeStr=boolean  PortDimensions=[6]  SampleTime=5.12820512820513e-07
  sch_ctr_36 : Inport  Port=4  OutDataTypeStr=fixdt(0, 6, 0)  SampleTime=1.38600138600139e-08
  Discrete-Time Integrator_reg : RateTransition  InitialCondition=double(0)  OutPortSampleTimeOpt=Multiple of input port sample time  OutPortSampleTimeMultiple=37
  Discrete-Time Integrator_reg_absorbed : Delay  DelayLength=0
  crp_temp_streamed : Subsystem
  in0_repeat : RateTransition  Integrity=off  Deterministic=off  OutPortSampleTimeOpt=Multiple of input port sample time  OutPortSampleTimeMultiple=1/37
  in3_repeat : RateTransition  Integrity=off  Deterministic=off  OutPortSampleTimeOpt=Multiple of input port sample time  OutPortSampleTimeMultiple=1/37
  ic : Outport  SampleTime=1.38600138600139e-08
  wires:
  Discrete-Time Integrator_reg_absorbed/1 -> in0_repeat/1
  Discrete-Time Integrator_reg/1 -> Discrete-Time Integrator_reg_absorbed/1
  crp_temp_streamed/2(out1) -> ic/1
  in0_repeat/1 -> crp_temp_streamed/1(in0)
  sch_ctr_36/1 -> crp_temp_streamed/5(enb_counter)
  is/1 -> crp_temp_streamed/4(in3)
  crp_temp_streamed/1(out0) -> Discrete-Time Integrator_reg/1
  in3_repeat/1 -> crp_temp_streamed/2(in1)
  vs/1 -> crp_temp_streamed/3(in2)
  G/1 -> in3_repeat/1

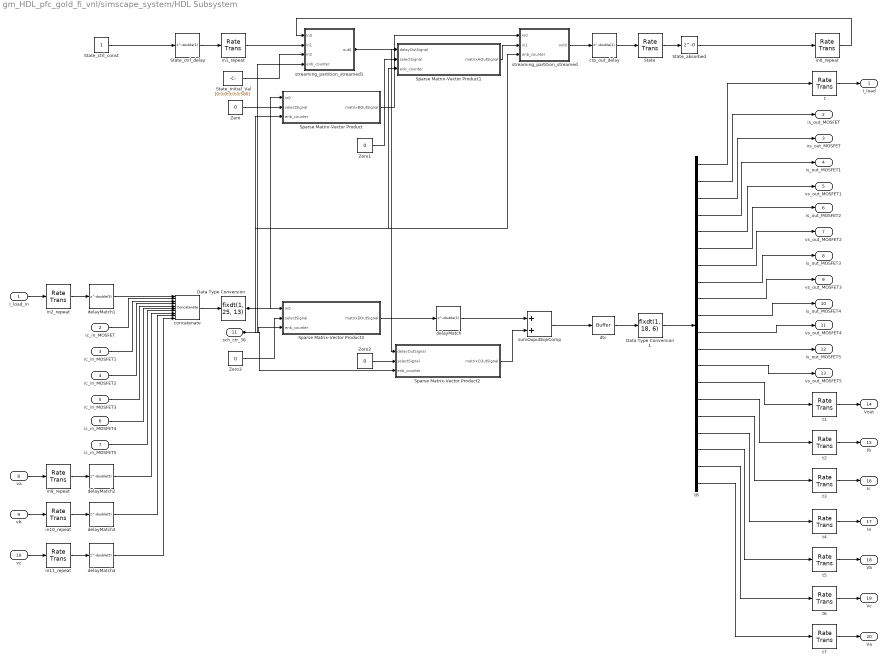
== system gm_HDL_pfc_gold_fi_vnl/simscape_system/HDL Subsystem ==
  I_load_in : Inport  OutDataTypeStr=fixdt(1, 18, 8)  PortDimensions=1  SampleTime=5.12820512820513e-07
  ic_in_MOSFET : Inport  Port=2  OutDataTypeStr=fixdt(1, 18, 8)  PortDimensions=1  SampleTime=1.38600138600139e-08
  ic_in_MOSFET1 : Inport  Port=3  OutDataTypeStr=fixdt(1, 18, 8)  PortDimensions=1  SampleTime=1.38600138600139e-08
  ic_in_MOSFET2 : Inport  Port=4  OutDataTypeStr=fixdt(1, 18, 8)  PortDimensions=1  SampleTime=1.38600138600139e-08
  ic_in_MOSFET3 : Inport  Port=5  OutDataTypeStr=fixdt(1, 18, 8)  PortDimensions=1  SampleTime=1.38600138600139e-08
  ic_in_MOSFET4 : Inport  Port=6  OutDataTypeStr=fixdt(1, 18, 8)  PortDimensions=1  SampleTime=1.38600138600139e-08
  ic_in_MOSFET5 : Inport  Port=7  OutDataTypeStr=fixdt(1, 18, 8)  PortDimensions=1  SampleTime=1.38600138600139e-08
  va : Inport  Port=8  OutDataTypeStr=fixdt(1, 18, 8)  PortDimensions=1  SampleTime=5.12820512820513e-07
  vb : Inport  Port=9  OutDataTypeStr=fixdt(1, 18, 8)  PortDimensions=1  SampleTime=5.12820512820513e-07
  vc : Inport  Port=10  OutDataTypeStr=fixdt(1, 18, 8)  PortDimensions=1  SampleTime=5.12820512820513e-07
  sch_ctr_36 : Inport  Port=11  OutDataTypeStr=fixdt(0, 6, 0)  SampleTime=1.38600138600139e-08
  Data Type Conversion : DataTypeConversion  OutDataTypeStr=fixdt(1, 25, 13)  SampleTime=1.38600138600139e-08  SaturateOnIntegerOverflow=off  RndMeth=Floor
  Data Type Conversion1 : DataTypeConversion  OutDataTypeStr=fixdt(1, 18, 6)  SampleTime=1.38600138600139e-08  SaturateOnIntegerOverflow=off  RndMeth=Floor
  Sparse Matrix-Vector Product : Subsystem
  Sparse Matrix-Vector Product1 : Subsystem
  Sparse Matrix-Vector Product2 : Subsystem
  Sparse Matrix-Vector Product3 : Subsystem
  State : RateTransition  InitialCondition=double(0)  OutPortSampleTimeOpt=Multiple of input port sample time  OutPortSampleTimeMultiple=37
  State_Initial_Val : Constant  Value=[0;0;0;0;0;0;580]  OutDataTypeStr=fixdt(1, 25, 13)  SampleTime=1.38600138600139e-08
  State_absorbed : Delay  DelayLength=0
  State_ctrl_const : Constant  OutDataTypeStr=boolean  SampleTime=5.12820512820513e-07
  State_ctrl_delay : Delay  DelayLength=double(1)  InitialCondition=0  SampleTime=5.12820512820513e-07
  Zero{,1..3} (4 alike) : Constant  Value=0  OutDataTypeStr=boolean  SampleTime=1.38600138600139e-08
  concatenate : Concatenate  NumInputs=10
  crp_out_delay : Delay  DelayLength=double(1)  InitialCondition=0  SampleTime=1.38600138600139e-08
  delayMatch : Delay  DelayLength=double(1)  InitialCondition=0  SampleTime=1.38600138600139e-08
  delayMatch{1..4} (4 alike) : Delay  DelayLength=double(5)  InitialCondition=0  SampleTime=1.38600138600139e-08
  dtc : hdlmdlgenlib/Buffer
  in0_repeat : RateTransition  Integrity=off  Deterministic=off  OutPortSampleTimeOpt=Multiple of input port sample time  OutPortSampleTimeMultiple=1/37
  in10_repeat : RateTransition  Integrity=off  Deterministic=off  OutPortSampleTimeOpt=Multiple of input port sample time  OutPortSampleTimeMultiple=1/37
  in11_repeat : RateTransition  Integrity=off  Deterministic=off  OutPortSampleTimeOpt=Multiple of input port sample time  OutPortSampleTimeMultiple=1/37
  in1_repeat : RateTransition  Integrity=off  Deterministic=off  OutPortSampleTimeOpt=Multiple of input port sample time  OutPortSampleTimeMultiple=1/37
  in2_repeat : RateTransition  Integrity=off  Deterministic=off  OutPortSampleTimeOpt=Multiple of input port sample time  OutPortSampleTimeMultiple=1/37
  in9_repeat : RateTransition  Integrity=off  Deterministic=off  OutPortSampleTimeOpt=Multiple of input port sample time  OutPortSampleTimeMultiple=1/37
  streaming_partition_streamed : Subsystem
  streaming_partition_streamed1 : Subsystem
  sumOuputEqnComp : Sum  OutDataTypeStr=fixdt(1, 25, 13)  SampleTime=1.38600138600139e-08
  t{,1..7} (8 alike) : RateTransition  InitialCondition=double(0)  OutPortSampleTimeOpt=Multiple of input port sample time  OutPortSampleTimeMultiple=37
  t8 : Demux  Outputs=20
  I_load : Outport  SampleTime=5.12820512820513e-07
  is_out_MOSFET : Outport  Port=2  SampleTime=1.38600138600139e-08
  vs_out_MOSFET : Outport  Port=3  SampleTime=1.38600138600139e-08
  is_out_MOSFET1 : Outport  Port=4  SampleTime=1.38600138600139e-08
  vs_out_MOSFET1 : Outport  Port=5  SampleTime=1.38600138600139e-08
  is_out_MOSFET2 : Outport  Port=6  SampleTime=1.38600138600139e-08
  vs_out_MOSFET2 : Outport  Port=7  SampleTime=1.38600138600139e-08
  is_out_MOSFET3 : Outport  Port=8  SampleTime=1.38600138600139e-08
  vs_out_MOSFET3 : Outport  Port=9  SampleTime=1.38600138600139e-08
  is_out_MOSFET4 : Outport  Port=10  SampleTime=1.38600138600139e-08
  vs_out_MOSFET4 : Outport  Port=11  SampleTime=1.38600138600139e-08
  is_out_MOSFET5 : Outport  Port=12  SampleTime=1.38600138600139e-08
  vs_out_MOSFET5 : Outport  Port=13  SampleTime=1.38600138600139e-08
  Vout : Outport  Port=14  SampleTime=5.12820512820513e-07
  Ib : Outport  Port=15  SampleTime=5.12820512820513e-07
  Ic : Outport  Port=16  SampleTime=5.12820512820513e-07
  Ia : Outport  Port=17  SampleTime=5.12820512820513e-07
  Vb : Outport  Port=18  SampleTime=5.12820512820513e-07
  Vc : Outport  Port=19  SampleTime=5.12820512820513e-07
  Va : Outport  Port=20  SampleTime=5.12820512820513e-07
  wires:
  t7/1 -> Va/1
  t6/1 -> Vc/1
  t4/1 -> Ia/1
  t3/1 -> Ic/1
  t2/1 -> Ib/1
  t1/1 -> Vout/1
  t/1 -> I_load/1
  t8/13 -> vs_out_MOSFET5/1
  t8/14 -> t1/1
  t8/11 -> vs_out_MOSFET4/1
  t8/12 -> is_out_MOSFET5/1
  in0_repeat/1 -> streaming_partition_streamed1/1(in0)
  t8/7 -> vs_out_MOSFET2/1
  t8/8 -> is_out_MOSFET3/1
  t8/5 -> vs_out_MOSFET1/1
  t8/6 -> is_out_MOSFET2/1
  t8/3 -> vs_out_MOSFET/1
  t8/1 -> t/1
  t8/2 -> is_out_MOSFET/1
  State_absorbed/1 -> in0_repeat/1
  State/1 -> State_absorbed/1
  dtc/1 -> Data Type Conversion1/1
  sumOuputEqnComp/1 -> dtc/1
  streaming_partition_streamed/1(out0) -> crp_out_delay/1
  t8/4 -> is_out_MOSFET1/1
  delayMatch/1 -> sumOuputEqnComp/1
  Zero2/1 -> Sparse Matrix-Vector Product2/2(selectSignal)
  Sparse Matrix-Vector Product2/1(matrixCOutSignal) -> sumOuputEqnComp/2
  t8/17 -> t4/1
  Sparse Matrix-Vector Product3/1(matrixDOutSignal) -> delayMatch/1
  t8/18 -> t5/1
  Zero1/1 -> Sparse Matrix-Vector Product1/2(selectSignal)
  streaming_partition_streamed1/1(out0) -> Sparse Matrix-Vector Product1/1(delayOutSignal), Sparse Matrix-Vector Product2/1(delayOutSignal)
  Zero3/1 -> Sparse Matrix-Vector Product3/2(selectSignal)
  sch_ctr_36/1 -> streaming_partition_streamed/3(enb_counter), Sparse Matrix-Vector Product1/3(enb_counter), Sparse Matrix-Vector Product/3(enb_counter), streaming_partition_streamed1/4(enb_counter), Sparse Matrix-Vector Product3/3(enb_counter), Sparse Matrix-Vector Product2/3(enb_counter)
  Data Type Conversion/1 -> Sparse Matrix-Vector Product3/1(in0), Sparse Matrix-Vector Product/1(in0)
  State_Initial_Val/1 -> streaming_partition_streamed1/3(in2)
  in1_repeat/1 -> streaming_partition_streamed1/2(in1)
  concatenate/1 -> Data Type Conversion/1
  State_ctrl_delay/1 -> in1_repeat/1
  delayMatch4/1 -> concatenate/10
  t8/19 -> t6/1
  delayMatch3/1 -> concatenate/9
  t8/20 -> t7/1
  delayMatch2/1 -> concatenate/8
  t8/9 -> vs_out_MOSFET3/1
  t8/10 -> is_out_MOSFET4/1
  ic_in_MOSFET5/1 -> concatenate/7
  Data Type Conversion1/1 -> t8/1
  ic_in_MOSFET2/1 -> concatenate/4
  ic_in_MOSFET1/1 -> concatenate/3
  ic_in_MOSFET4/1 -> concatenate/6
  delayMatch1/1 -> concatenate/1
  State_ctrl_const/1 -> State_ctrl_delay/1
  ic_in_MOSFET3/1 -> concatenate/5
  in10_repeat/1 -> delayMatch3/1
  in2_repeat/1 -> delayMatch1/1
  t8/15 -> t2/1
  t8/16 -> t3/1
  vc/1 -> in11_repeat/1
  ic_in_MOSFET/1 -> concatenate/2
  t5/1 -> Vb/1
  vb/1 -> in10_repeat/1
  Zero/1 -> Sparse Matrix-Vector Product/2(selectSignal)
  Sparse Matrix-Vector Product1/1(matrixAOutSignal) -> streaming_partition_streamed/2(in1)
  in9_repeat/1 -> delayMatch2/1
  va/1 -> in9_repeat/1
  Sparse Matrix-Vector Product/1(matrixBOutSignal) -> streaming_partition_streamed/1(in0)
  in11_repeat/1 -> delayMatch4/1
  I_load_in/1 -> in2_repeat/1
  crp_out_delay/1 -> State/1

== system gm_HDL_pfc_gold_fi_vnl/simscape_system_vnl/FET_CTRL ==
  vs : Inport  OutDataTypeStr=fixdt(1,18,6)
  is : Inport  Port=2  OutDataTypeStr=fixdt(1,18,6)
  G : Inport  Port=3
  Constant : Constant  Value=-.7  OutDataTypeStr=fixdt(1,18,17)  SampleTime=-1
  Discrete-Time Integrator : DiscreteIntegrator  IntegratorMethod=Accumulation: Forward Euler  gainval=1/s  SampleTime=-1  OutDataTypeStr=fixdt(1,18,8)  ICPrevOutput=DiscIntNeverNeededParam  ICPrevScaledInput=DiscIntNeverNeededParam
  Equal : RelationalOperator  OutDataTypeStr=boolean  RndMeth=Simplest  InputSameDT=off
  Gain1 : Gain  Gain=-1  OutDataTypeStr=fixdt(1,18,12)
  Gain3 : Gain  Gain=Gs  OutDataTypeStr=fixdt(1,18,12)
  Multiply-Add : hdlsllib/HDL Operations/Multiply-Add  Function=c+(a.*b)  datatype=fixdt(1,18,12)  DoSatur=off  FMA=off
  OR : Logic  Operator=OR  IconShape=distinctive  AllPortsSameDT=off  OutDataTypeStr=boolean
  Subtract : Sum  Inputs=+-  OutDataTypeStr=fixdt(1,18,12)
  Subtract1 : Sum  Inputs=+-  OutDataTypeStr=fixdt(1,18,11)
  ic : Outport
  wires:
  vs/1 -> Equal/2, Gain3/1
  G/1 -> OR/1
  is/1 -> Gain1/1
  Multiply-Add/1 -> Subtract/1
  Gain1/1 -> Subtract1/1  "on"
  Discrete-Time Integrator/1 -> ic/1, Subtract/2  "ic"
  Subtract/1 -> Discrete-Time Integrator/1
  Equal/1 -> OR/2
  Constant/1 -> Equal/1
  Gain3/1 -> Subtract1/2, Multiply-Add/3
  Subtract1/1 -> Multiply-Add/1
  OR/1 -> Multiply-Add/2
